simulink model "drive"  (R2022b)
settings: Solver=VariableStepAuto  StartTime=0.0  StopTime=10  RelTol=1e-3
libraries: simulink_extras x4
settings Model: PacingRate=0.890000  Creator=Administrator  LastModifiedBy=Administrator

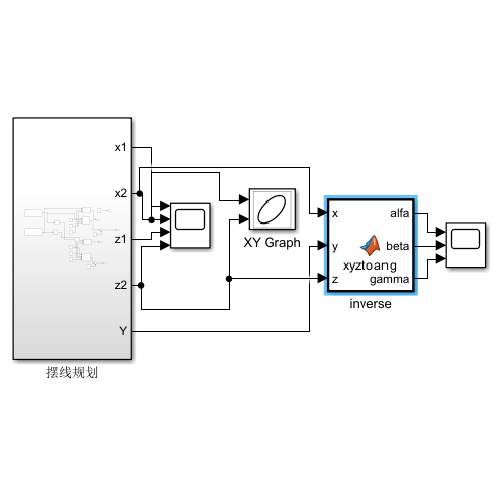
[thumbnail: Simulink's stored preview of the top-level diagram]
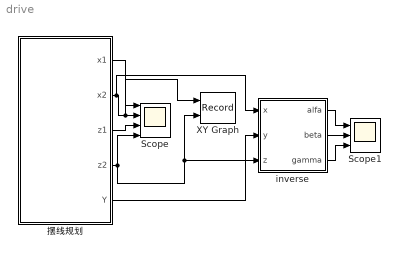
== system drive ==
  Scope : Scope  NumInputPorts=4
  Scope1 : Scope  NumInputPorts=3
  XY Graph : Record  FileSettingsInternal="{\"entries\":[{\"content\":{\"excelSettings\":{\"content\":{},\"type\":\"Streamout.ExcelSettings\"}},\"type\":\"Streamout.FileSettingStorage\",\"uuid\":\"e4057471-3260-48cd-bdf4-47e10ce90d70\"}],\"packageUris\":[\"http://schema.mathworks.com/mf0/streamout_blocks/R2020a\"],\"version\":\"1.0\"}"  Layout=[1 1]  SignalsInternal="{\"entries\":[{\"content\":{\"signals\":[{\"content\":{\"blockPath\":[\"drive/XY Graph\"],\"channel\":[],\"dimensions\":[1],\"domain\":\"drive/XY Graph\",\"lineColor\":\"#a2142f\",\"plots\":[1],\"port\":1,\"sid\":[\"\"],\"signalID\":36,\"signalName\":\"摆线规划:2\"},\"type\":\"RecordBlkView.Signal\",\"uuid\":\"2e63d6af-6ebe-4c5c-b3b5-8981d4e213b3\"},{\"content\":{\"blockPath\":[\"drive/XY Graph\"],\"channel\":[],\"dimensions\":[1],\"domain\":\"drive/XY Graph\",\"lineColor\":\"#139fff\",\"plots\":[1],\"port\":2,\"sid\":[\"\"],\"signalID\":40,\"signalName\":\"摆线规划:4\"},\"type\":\"RecordBlkView.Signal\",\"uuid\":\"96254a20-061c-4f52-8165-9b07dd72a1a5\"}]},\"type\":\"RecordBlkView.InputSignals\",\"uuid\":\"8ff8d1e1-72ba-4ce4-9b96-e7de07653a36\"}],\"packageUris\":[\"http://schema.mathworks.com/mf0/streamout_blocks/R2020a\"],\"version\":\"1.0\"}"  VisualizationBindings="{\"xyplotplugin\":{\"info\":[{\"series\":[{\"bindingParametersList\":[{\"parameter\":\"X-Axis\",\"signalID\":36,\"signalName\":\"摆线规划:2\"},{\"parameter\":\"Y-Axis\",\"signalID\":40,\"signalName\":\"摆线规划:4\"}],\"seriesID\":57678}],\"subplotID\":1}]}}"  CompatibilityTag=XY
  inverse : MATLAB Function  TreatAsAtomicUnit=on
  摆线规划 : Subsystem
  wires:
  摆线规划/1(x1) -> Scope/1
  摆线规划/2(x2) -> inverse/1(x), XY Graph/1, Scope/2
  摆线规划/3(z1) -> Scope/3
  摆线规划/4(z2) -> XY Graph/2, inverse/3(z), Scope/4
  摆线规划/5(Y) -> inverse/2(y)
  inverse/1(alfa) -> Scope1/1
  inverse/2(beta) -> Scope1/2
  inverse/3(gamma) -> Scope1/3

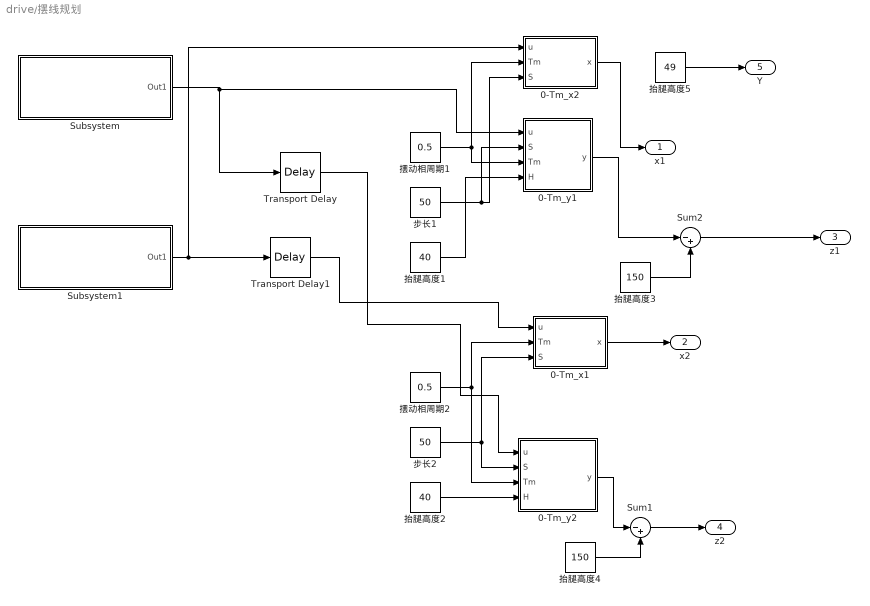
== system drive/摆线规划 ==
  0-Tm_x1 : MATLAB Function  TreatAsAtomicUnit=on
  0-Tm_x2 : MATLAB Function  TreatAsAtomicUnit=on
  0-Tm_y1 : MATLAB Function  TreatAsAtomicUnit=on
  0-Tm_y2 : MATLAB Function  TreatAsAtomicUnit=on
  Subsystem : Subsystem
  Subsystem1 : Subsystem
  Sum1 : Sum  Inputs=|-+
  Sum2 : Sum  Inputs=|-+
  Transport Delay : TransportDelay  DelayTime=0.5
  Transport Delay1 : TransportDelay  DelayTime=0.5
  抬腿高度1 : Constant  Value=40
  抬腿高度2 : Constant  Value=40
  抬腿高度3 : Constant  Value=150
  抬腿高度4 : Constant  Value=150
  抬腿高度5 : Constant  Value=49
  摆动相周期1 : Constant  Value=0.5
  摆动相周期2 : Constant  Value=0.5
  步长1 : Constant  Value=50
  步长2 : Constant  Value=50
  x1 : Outport  VectorParamsAs1DForOutWhenUnconnected=off
  x2 : Outport  Port=2  VectorParamsAs1DForOutWhenUnconnected=off
  z1 : Outport  Port=3  VectorParamsAs1DForOutWhenUnconnected=off
  z2 : Outport  Port=4  VectorParamsAs1DForOutWhenUnconnected=off
  Y : Outport  Port=5  VectorParamsAs1DForOutWhenUnconnected=off
  wires:
  Sum2/1 -> z1/1
  0-Tm_y1/1(y) -> Sum2/1
  抬腿高度3/1 -> Sum2/2
  Sum1/1 -> z2/1
  0-Tm_y2/1(y) -> Sum1/1
  抬腿高度4/1 -> Sum1/2
  Transport Delay1/1 -> 0-Tm_x1/1(u)
  Subsystem1/1(Out1) -> 0-Tm_x2/1(u), Transport Delay1/1
  0-Tm_x1/1(x) -> x2/1
  摆动相周期2/1 -> 0-Tm_y2/3(Tm), 0-Tm_x1/2(Tm)
  0-Tm_x2/1(x) -> x1/1
  步长2/1 -> 0-Tm_y2/2(S), 0-Tm_x1/3(S)
  步长1/1 -> 0-Tm_x2/3(S), 0-Tm_y1/2(S)
  抬腿高度1/1 -> 0-Tm_y1/4(H)
  摆动相周期1/1 -> 0-Tm_x2/2(Tm), 0-Tm_y1/3(Tm)
  Subsystem/1(Out1) -> Transport Delay/1, 0-Tm_y1/1(u)
  抬腿高度2/1 -> 0-Tm_y2/4(H)
  Transport Delay/1 -> 0-Tm_y2/1(u)
  抬腿高度5/1 -> Y/1

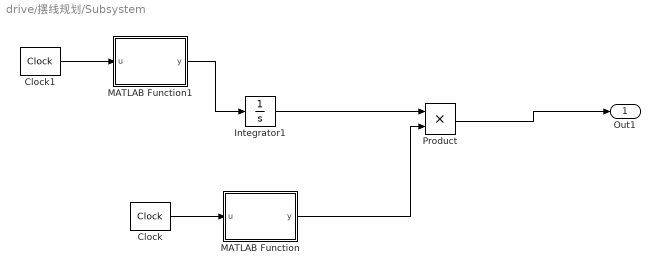
== system drive/摆线规划/Subsystem ==
  Clock : simulink_extras/Flip Flops/Clock  period=1
  Clock1 : simulink_extras/Flip Flops/Clock  period=0.5
  Integrator1 : Integrator
  MATLAB Function : MATLAB Function  TreatAsAtomicUnit=on
  MATLAB Function1 : MATLAB Function  TreatAsAtomicUnit=on
  Product : Product
  Out1 : Outport  VectorParamsAs1DForOutWhenUnconnected=off
  wires:
  Product/1 -> Out1/1
  Integrator1/1 -> Product/1
  Clock/1 -> MATLAB Function/1(u)
  MATLAB Function/1(y) -> Product/2
  Clock1/1 -> MATLAB Function1/1(u)
  MATLAB Function1/1(y) -> Integrator1/1

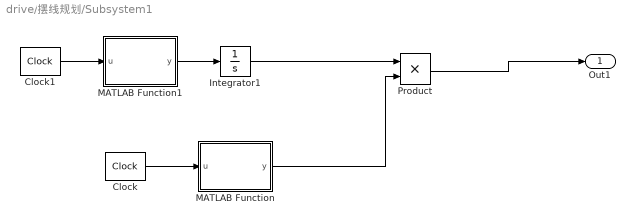
== system drive/摆线规划/Subsystem1 ==
  Clock : simulink_extras/Flip Flops/Clock  period=2
  Clock1 : simulink_extras/Flip Flops/Clock  period=1
  Integrator1 : Integrator
  MATLAB Function : MATLAB Function  TreatAsAtomicUnit=on
  MATLAB Function1 : MATLAB Function  TreatAsAtomicUnit=on
  Product : Product
  Out1 : Outport  VectorParamsAs1DForOutWhenUnconnected=off
  wires:
  Product/1 -> Out1/1
  Integrator1/1 -> Product/1
  Clock/1 -> MATLAB Function/1(u)
  MATLAB Function/1(y) -> Product/2
  Clock1/1 -> MATLAB Function1/1(u)
  MATLAB Function1/1(y) -> Integrator1/1

== matlab function drive/inverse ==
  data: x input; alfa output; y input; z input; beta output; gamma output
function [alfa, beta, gamma]=xyztoang(x, y, z)
    h_up=49.0;
    h_mid=125.5899;
    h_low=116.0+20;
    dyz=sqrt(y.^2+z.^2);
    lyz=sqrt(dyz.^2-h_up.^2);
    gamma_yz=-atan(y./z);
    gamma_h_offset=-atan(h_up./lyz);
    gamma=gamma_yz-gamma_h_offset;
    lxzp=sqrt(lyz.^2+x.^2);
    n=(lxzp.^2-h_low^2-h_mid.^2)/(2*h_mid);
    beta=-acos(n/h_low);
    alfa_xzp=-atan(x/lyz);
    alfa_off=acos((h_mid+n)/lxzp);
    alfa=(alfa_xzp+alfa_off);
end

== matlab function drive/摆线规划/0-Tm_x1 ==
  data: u input; x output; Tm input; S input
function x = fcn(u,Tm,S)


if u>0
   
    x =S*(u/Tm-1/(2*pi)*sin(2*pi*u/Tm));
else 
    u=-u;
    x =S*(u/Tm-1/(2*pi)*sin(2*pi*u/Tm));
end

== matlab function drive/摆线规划/0-Tm_x2 ==
  data: u input; x output; Tm input; S input
function x = fcn(u,Tm,S)

if u>0
    x =S*(u/Tm-1/(2*pi)*sin(2*pi*u/Tm));
else 
    u=-u;
     x =S*(u/Tm-1/(2*pi)*sin(2*pi*u/Tm));
end

== matlab function drive/摆线规划/0-Tm_y1 ==
  data: u input; y output; S input; Tm input; H input
function y = fcn(u,S,Tm,H)

n=4;
if u>0
    y=2*H*(u/Tm-1/(n*pi)*sin(n*pi*u/Tm)).*(u>=0&u<Tm/2)+2*H*(1-u/Tm+1/(n*pi)*sin(n*pi*u/Tm)).*(u>=Tm/2&u<Tm);;
else 
    y=0;
end

== matlab function drive/摆线规划/0-Tm_y2 ==
  data: u input; y output; S input; Tm input; H input
function y = fcn(u,S,Tm,H)

n=4;
if u>0
    y=2*H*(u/Tm-1/(n*pi)*sin(n*pi*u/Tm)).*(u>=0&u<Tm/2)+2*H*(1-u/Tm+1/(n*pi)*sin(n*pi*u/Tm)).*(u>=Tm/2&u<Tm);;
else 
    y=0;
end

== matlab function drive/摆线规划/Subsystem/MATLAB Function ==
  data: u input; y output
function y = fcn(u)
if u==0
    y = -1;
else
    y=1;
end
end

== matlab function drive/摆线规划/Subsystem/MATLAB Function1 ==
  data: u input; y output
function y = fcn(u)
if u==0
    y = -1;
else
    y=1;
end
end

== matlab function drive/摆线规划/Subsystem1/MATLAB Function ==
  data: u input; y output
function y = fcn(u)
if u==0
    y = -1;
else
    y=1;
end
end

== matlab function drive/摆线规划/Subsystem1/MATLAB Function1 ==
  data: u input; y output
function y = fcn(u)
if u==0
    y = -1;
else
    y=1;
end
end
